simulink model "motion_with_control_two_robots"  (R2025a)
settings: Solver=FixedStepDiscrete  StartTime=0.0  StopTime=inf  FixedStep=0.01  RelTol=1e-3  EnableMultiTasking=on
PreLoadFcn:
  | frs = FrankaRobotSettings;
libraries: franka_simulink x2
settings Model: SimulationMode=external  ExtModeTrigDuration=10000  Creator=vasi_ko  LastModifiedBy=kvasios
settings SolverCC: ConcurrentTasks=on  AlgebraicLoopSolver=TrustRegion  AutoInsertRateTranBlk=on
settings DataIOCC: LimitDataPoints=on  SaveFormat=Array  ReturnWorkspaceOutputs=off
settings OptimizationCC: EnhancedBackFolding=on  PassReuseOutputArgsAs=Individual arguments  ZeroExternalMemoryAtStartup=off  ZeroInternalMemoryAtStartup=off  MaxStackSize=200000  OptimizeBlockOrder=speed  DifferentSizesBufferReuse=on  OptimizationCustomize=off  EfficientTunableParamExpr=on
settings DebuggingCC: SolverPrmCheckMsg=warning  ParameterTunabilityLossMsg=error  UnconnectedInputMsg=warning  UnconnectedOutputMsg=warning  UnconnectedLineMsg=warning  SFUnexpectedBacktrackingDiag=warning  SFNoUnconditionalDefaultTransitionDiag=warning  SFExecutionAtInitializationDiag=none  ArithmeticOperatorsInVariantConditions=warning
settings HardwareCC: ProdBitPerLong=64.0  ProdLargestAtomicInteger=LongLong  ProdLargestAtomicFloat=Double  ProdLongLongMode=on  ProdHWDeviceType=ARM Compatible->ARM Cortex-A (64-bit)
settings ModelReferenceCC: EnableRefExpFcnMdlSchedulingChecks=on  PropagateSignalLabelsOutOfModel=off
settings SFSimCC: SimUseLocalCustomCode=off  MATLABDynamicMemAlloc=off  CustomCodeUndefinedFunction=UseInterfaceOnly  SimTargetLang=C++  SimDLTargetLibrary=mkl-dnn
settings RTWCC: SystemTargetFile=ert.tlc  HardwareBoard=NVIDIA Jetson  TLCOptions="-aInlineSetEventsForThisBaseRateFcn=TLC_FALSE -aSuppressMultiTaskScheduler=TLC_FALSE  -aRateBasedStepFcn=0"  TemplateMakefile=ert_default_tmf  RTWVerbose=off  RTWUseLocalCustomCode=off  BuildConfiguration=Faster Runs  TargetLang=C++  GPUComputeCapability=3.5  DLArmComputeVersion=19.05  Description=Embedded Coder
settings CodeAppCC: ForceParamTrailComments=on  IgnoreCustomStorageClasses=off  OperatorAnnotations=on  SimulinkDataObjDesc=on  SFDataObjDesc=on  InsertBlockDesc=on
settings ERTTargetCC: ExtModeTransport=2.0  InlinedParameterPlacement=Hierarchical  RootIOFormat=Structure reference  TargetLangStandard=C++14 (ISO)
settings ConfigComp: CovMetricSettings=dw  CovSaveCumulativeToWorkspaceVar=on  CovSaveSingleToWorkspaceVar=on  CovExternalEMLEnable=off  CovSFcnEnable=off

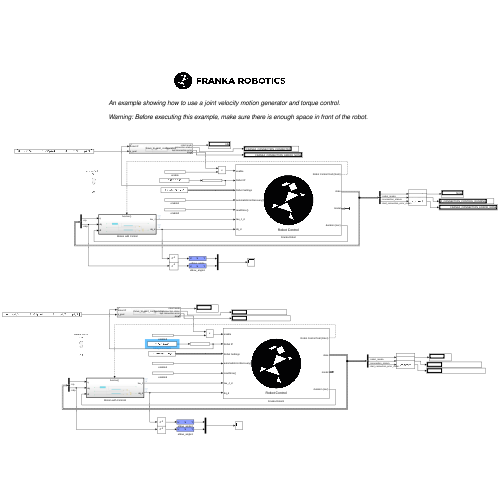
[thumbnail: Simulink's stored preview of the top-level diagram]
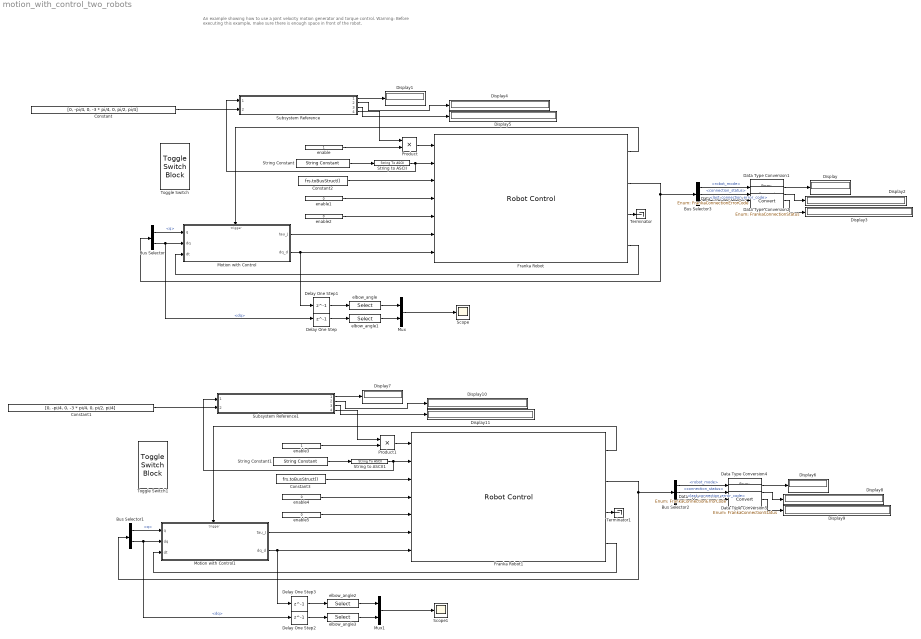
== system motion_with_control_two_robots ==
  note: An example showing how to use a joint velocity motion generator and torque control.
      |
      | Warning: Before executing this example, make sure there is enough space in front of the robot.
  Bus Selector : BusSelector  OutputSignals=q,dq
  Bus Selector1 : BusSelector  OutputSignals=q,dq
  Bus Selector2 : BusSelector  OutputSignals=robot_mode,connection_status,last_connection_error_code
  Bus Selector3 : BusSelector  OutputSignals=robot_mode,connection_status,last_connection_error_code
  Constant : Constant  Value=[0, -pi/4, 0, -3 * pi/4, 0, pi/2, pi/4]
  Constant1 : Constant  Value=[0, -pi/4, 0, -3 * pi/4, 0, pi/2, pi/4]
  Constant2 : Constant  Value=frs.toBusStruct()  OutDataTypeStr=Bus: FrankaRobotSettingsBus
  Constant3 : Constant  Value=frs.toBusStruct()  OutDataTypeStr=Bus: FrankaRobotSettingsBus
  Data Type Conversion1 : DataTypeConversion  OutDataTypeStr=Enum: FrankaRobotModes  SaturateOnIntegerOverflow=off  RndMeth=Floor
  Data Type Conversion2 : DataTypeConversion  OutDataTypeStr=Enum: FrankaConnectionStatus  SaturateOnIntegerOverflow=off  RndMeth=Floor
  Data Type Conversion3 : DataTypeConversion  OutDataTypeStr=Enum: FrankaConnectionErrorCode  SaturateOnIntegerOverflow=off  RndMeth=Floor
  Data Type Conversion4 : DataTypeConversion  OutDataTypeStr=Enum: FrankaRobotModes  SaturateOnIntegerOverflow=off  RndMeth=Floor
  Data Type Conversion5 : DataTypeConversion  OutDataTypeStr=Enum: FrankaConnectionStatus  SaturateOnIntegerOverflow=off  RndMeth=Floor
  Data Type Conversion6 : DataTypeConversion  OutDataTypeStr=Enum: FrankaConnectionErrorCode  SaturateOnIntegerOverflow=off  RndMeth=Floor
  Delay One Step{,1..3} (4 alike) : Delay  DelayLength=1
  Display{,1..11} (12 alike) : Display
  Franka Robot : franka_simulink/Robot Control  control_mode=Torques + Joint Velocities  rt_priority=80  rt_cpu_affinity=-1  rt_lock_memory=off
      settings: SourceProductName=Franka Robotics Simulink Support Package
  Franka Robot1 : franka_simulink/Robot Control  control_mode=Torques + Joint Velocities  rt_priority=80  rt_cpu_affinity=-1  rt_lock_memory=off
      settings: SourceProductName=Franka Robotics Simulink Support Package
  Motion with Control : Subsystem  TreatAsAtomicUnit=on
      settings: RTWSystemCode=Nonreusable function
  Motion with Control1 : Subsystem  TreatAsAtomicUnit=on
      settings: RTWSystemCode=Nonreusable function
  Mux : Mux  Inputs=2
  Mux1 : Mux  Inputs=2
  Product : Product
  Product1 : Product
  Scope : Scope
      settings: ActiveDisplayYMinimum=-0.68593897081558164  ActiveDisplayYMaximum=0.68922481990277773
  Scope1 : Scope
      settings: ActiveDisplayYMinimum=-0.68593897081558164  ActiveDisplayYMaximum=0.68922481990277773
  String Constant : StringConstant  String="\"172.16.0.2\""
  String Constant1 : StringConstant  String="\"172.16.0.3\""
  String to ASCII : StringToASCII  OutputVectorSize=16
  String to ASCII1 : StringToASCII  OutputVectorSize=16
  Subsystem Reference : Subsystem  ReferencedSubsystem=move_to_joint_configuration
  Subsystem Reference1 : Subsystem  ReferencedSubsystem=move_to_joint_configuration
  Terminator : Terminator
  Terminator1 : Terminator
  Toggle Switch : ToggleSwitchBlock
  Toggle Switch1 : ToggleSwitchBlock
  elbow_angle{,1..3} (4 alike) : Selector  InputPortWidth=7  IndexOptions=Index vector (dialog)  Indices=4  OutputSizes=1
  enable : Constant  SampleTime=-1
  enable{1..2,4..5} (4 alike) : Constant  Value=0  SampleTime=-1
  enable3 : Constant  SampleTime=-1
  wires:
  String to ASCII/1 -> Subsystem Reference/1, Franka Robot/2
  String Constant/1 -> String to ASCII/1
  Franka Robot/1 -> Motion with Control/Trigger
  Bus Selector/1 -> Motion with Control/1(q)  "<q>"
  Bus Selector/2 -> Delay One Step/1, Motion with Control/2(dq)  "<dq>"
  Franka Robot/4 -> Motion with Control/3(dt)
  Franka Robot/3 -> Terminator/1
  Constant2/1 -> Franka Robot/3
  Product/1 -> Franka Robot/1
  enable/1 -> Product/2
  Motion with Control/1(tau_J) -> Franka Robot/6
  enable1/1 -> Franka Robot/4
  enable2/1 -> Franka Robot/5
  Subsystem Reference/1 -> Display1/1
  Motion with Control/2(dq_d) -> Delay One Step1/1, Franka Robot/7
  elbow_angle/1 -> Mux/1
  elbow_angle1/1 -> Mux/2
  Mux/1 -> Scope/1
  Delay One Step/1 -> elbow_angle1/1
  Delay One Step1/1 -> elbow_angle/1
  Constant/1 -> Subsystem Reference/2
  Subsystem Reference/4 -> Product/1
  Subsystem Reference/2 -> Display4/1
  Subsystem Reference/3 -> Display5/1
  Bus Selector3/2 -> Data Type Conversion2/1  "<connection_status>"
  Data Type Conversion1/1 -> Display/1
  Franka Robot/2 -> Bus Selector3/1, Bus Selector/1
  Bus Selector3/1 -> Data Type Conversion1/1  "<robot_mode>"
  Data Type Conversion3/1 -> Display3/1
  Data Type Conversion2/1 -> Display2/1
  Bus Selector3/3 -> Data Type Conversion3/1  "<last_connection_error_code>"
  Bus Selector2/3 -> Data Type Conversion6/1  "<last_connection_error_code>"
  Data Type Conversion5/1 -> Display8/1
  Data Type Conversion6/1 -> Display9/1
  Bus Selector2/1 -> Data Type Conversion4/1  "<robot_mode>"
  Franka Robot1/2 -> Bus Selector1/1, Bus Selector2/1
  Data Type Conversion4/1 -> Display6/1
  Bus Selector2/2 -> Data Type Conversion5/1  "<connection_status>"
  Subsystem Reference1/3 -> Display11/1
  Subsystem Reference1/2 -> Display10/1
  Subsystem Reference1/4 -> Product1/1
  Constant1/1 -> Subsystem Reference1/2
  Delay One Step3/1 -> elbow_angle2/1
  Delay One Step2/1 -> elbow_angle3/1
  Mux1/1 -> Scope1/1
  elbow_angle3/1 -> Mux1/2
  elbow_angle2/1 -> Mux1/1
  Motion with Control1/2(dq_d) -> Franka Robot1/7, Delay One Step3/1
  Subsystem Reference1/1 -> Display7/1
  enable5/1 -> Franka Robot1/5
  enable4/1 -> Franka Robot1/4
  Motion with Control1/1(tau_J) -> Franka Robot1/6
  enable3/1 -> Product1/2
  Product1/1 -> Franka Robot1/1
  Constant3/1 -> Franka Robot1/3
  Franka Robot1/3 -> Terminator1/1
  Franka Robot1/4 -> Motion with Control1/3(dt)
  Bus Selector1/2 -> Motion with Control1/2(dq), Delay One Step2/1  "<dq>"
  Bus Selector1/1 -> Motion with Control1/1(q)  "<q>"
  Franka Robot1/1 -> Motion with Control1/Trigger
  String Constant1/1 -> String to ASCII1/1
  String to ASCII1/1 -> Franka Robot1/2, Subsystem Reference1/1

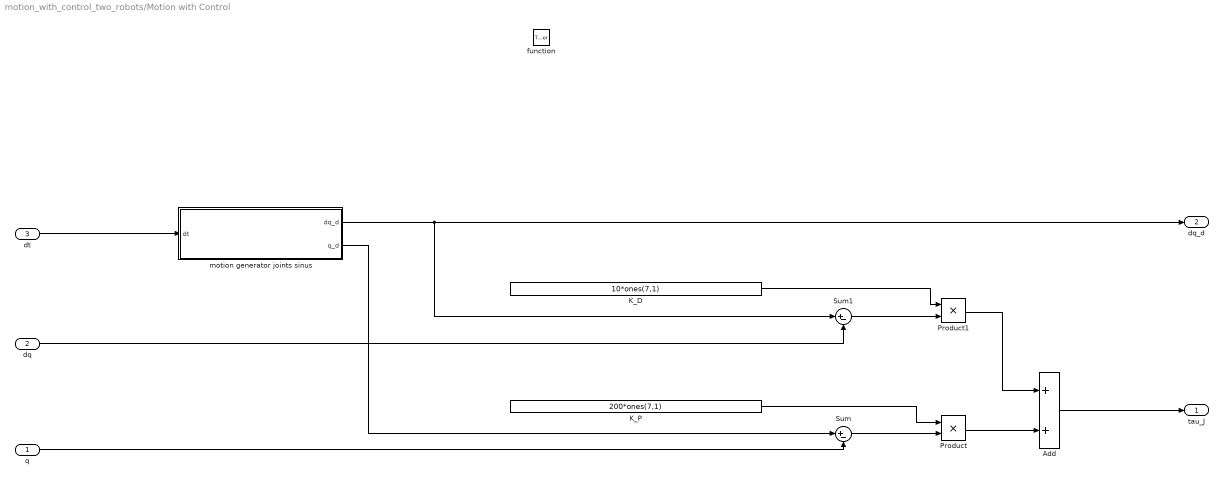
== system motion_with_control_two_robots/Motion with Control ==
  q : Inport
  dq : Inport  Port=2
  dt : Inport  Port=3
  function : TriggerPort  TriggerType=function-call  VariantControl=(inherit)  SampleTime=0.001
  Add : Sum
  K_D : Constant  Value=10*ones(7,1)  VectorParams1D=off  SampleTime=-1
  K_P : Constant  Value=200*ones(7,1)  VectorParams1D=off  SampleTime=-1
  Product : Product
  Product1 : Product
  Sum : Sum  Inputs=|+-
  Sum1 : Sum  Inputs=|+-
  motion generator joints sinus : Subsystem
      mask Display:
      | pos = get_param(gcb, 'Position');
      | width = pos(3) - pos(1);
      | x = [0:width];
      | y = sin(x/180*pi);
      | % Parameters 'm' and 'b' must be defined in 'Parameters & Dialog' pane.
      | plot(x,y );
      | 
      | port_label('output',1,'dq_d');
      | port_label('output',2,'q_d');
  tau_J : Outport  VectorParamsAs1DForOutWhenUnconnected=off
  dq_d : Outport  Port=2  VectorParamsAs1DForOutWhenUnconnected=off
  wires:
  Product1/1 -> Add/1
  Sum1/1 -> Product1/2
  dq/1 -> Sum1/2
  Product/1 -> Add/2
  Sum/1 -> Product/2
  K_D/1 -> Product1/1
  q/1 -> Sum/2
  K_P/1 -> Product/1
  dt/1 -> motion generator joints sinus/1(dt)
  motion generator joints sinus/1(dq_d) -> dq_d/1, Sum1/1
  motion generator joints sinus/2(q_d) -> Sum/1
  Add/1 -> tau_J/1

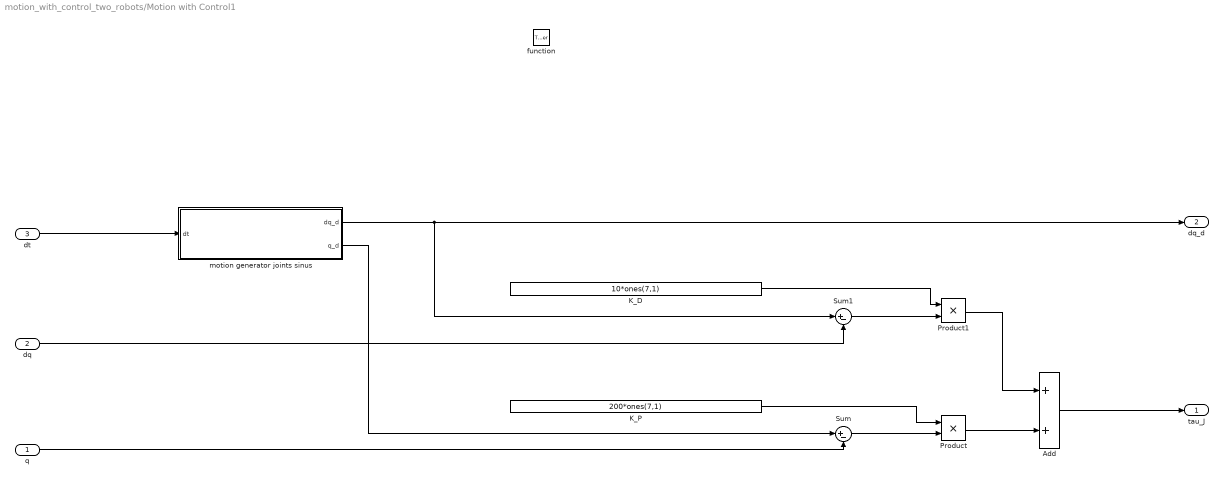
== system motion_with_control_two_robots/Motion with Control1 ==
  q : Inport
  dq : Inport  Port=2
  dt : Inport  Port=3
  function : TriggerPort  TriggerType=function-call  VariantControl=(inherit)  SampleTime=0.001
  Add : Sum
  K_D : Constant  Value=10*ones(7,1)  VectorParams1D=off  SampleTime=-1
  K_P : Constant  Value=200*ones(7,1)  VectorParams1D=off  SampleTime=-1
  Product : Product
  Product1 : Product
  Sum : Sum  Inputs=|+-
  Sum1 : Sum  Inputs=|+-
  motion generator joints sinus : Subsystem
      mask Display:
      | pos = get_param(gcb, 'Position');
      | width = pos(3) - pos(1);
      | x = [0:width];
      | y = sin(x/180*pi);
      | % Parameters 'm' and 'b' must be defined in 'Parameters & Dialog' pane.
      | plot(x,y );
      | 
      | port_label('output',1,'dq_d');
      | port_label('output',2,'q_d');
  tau_J : Outport  VectorParamsAs1DForOutWhenUnconnected=off
  dq_d : Outport  Port=2  VectorParamsAs1DForOutWhenUnconnected=off
  wires:
  Add/1 -> tau_J/1
  motion generator joints sinus/2(q_d) -> Sum/1
  motion generator joints sinus/1(dq_d) -> Sum1/1, dq_d/1
  dt/1 -> motion generator joints sinus/1(dt)
  K_P/1 -> Product/1
  q/1 -> Sum/2
  K_D/1 -> Product1/1
  Sum/1 -> Product/2
  Product/1 -> Add/2
  dq/1 -> Sum1/2
  Sum1/1 -> Product1/2
  Product1/1 -> Add/1

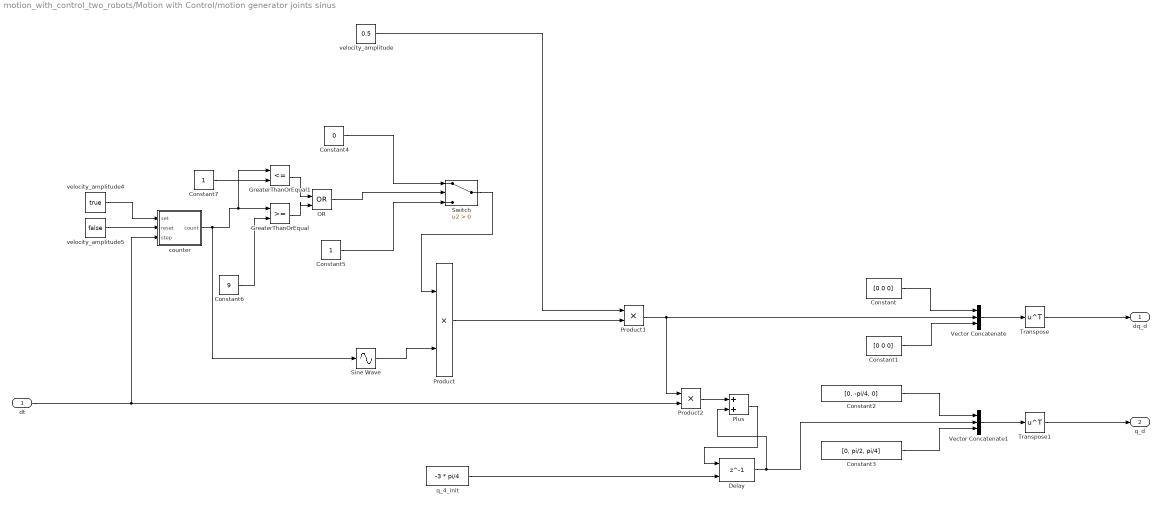
== system motion_with_control_two_robots/Motion with Control/motion generator joints sinus ==
  dt : Inport
  Constant : Constant  Value=[0 0 0]  VectorParams1D=off
  Constant1 : Constant  Value=[0 0 0]  VectorParams1D=off
  Constant2 : Constant  Value=[0, -pi/4, 0]  VectorParams1D=off
  Constant3 : Constant  Value=[0, pi/2, pi/4]  VectorParams1D=off
  Constant4 : Constant  Value=0
  Constant5 : Constant
  Constant6 : Constant  Value=9
  Constant7 : Constant
  Delay : Delay  DelayLength=1  InitialConditionSource=Input port
      settings: InputPortMap=u0,p4
  GreaterThanOrEqual : RelationalOperator  OutDataTypeStr=boolean  RndMeth=Simplest  InputSameDT=off
  GreaterThanOrEqual1 : RelationalOperator  Operator=<=  OutDataTypeStr=boolean  RndMeth=Simplest  InputSameDT=off
  OR : Logic  Operator=OR  IconShape=distinctive  AllPortsSameDT=off  OutDataTypeStr=boolean
  Plus : Sum
  Product : Product
  Product1 : Product
  Product2 : Product
  Sine Wave : Sin  TimeSource=Use external signal  Frequency=pi  Phase=pi
  Switch : Switch  Criteria=u2 > Threshold  SaturateOnIntegerOverflow=off  InputSameDT=off
  Transpose : Math  Operator=transpose
  Transpose1 : Math  Operator=transpose
  Vector Concatenate : Concatenate  NumInputs=3
  Vector Concatenate1 : Concatenate  NumInputs=3
  counter : Subsystem
  q_4_init : Constant  Value=-3 * pi/4  VectorParams1D=off
  velocity_amplitude : Constant  Value=0.5  VectorParams1D=off
  velocity_amplitude4 : Constant  Value=true  VectorParams1D=off
  velocity_amplitude5 : Constant  Value=false  VectorParams1D=off
  dq_d : Outport  VectorParamsAs1DForOutWhenUnconnected=off
  q_d : Outport  Port=2  VectorParamsAs1DForOutWhenUnconnected=off
  wires:
  Constant1/1 -> Vector Concatenate/3
  Constant/1 -> Vector Concatenate/1
  Product/1 -> Product1/2
  Sine Wave/1 -> Product/2
  velocity_amplitude/1 -> Product1/1
  Product1/1 -> Vector Concatenate/2, Product2/1
  Constant3/1 -> Vector Concatenate1/3
  Constant2/1 -> Vector Concatenate1/1
  q_4_init/1 -> Delay/2
  Delay/1 -> Vector Concatenate1/2, Plus/2
  Plus/1 -> Delay/1
  Product2/1 -> Plus/1
  Vector Concatenate/1 -> Transpose/1
  Vector Concatenate1/1 -> Transpose1/1
  Transpose/1 -> dq_d/1
  Transpose1/1 -> q_d/1
  velocity_amplitude4/1 -> counter/1(set)
  velocity_amplitude5/1 -> counter/2(reset)
  dt/1 -> counter/3(step), Product2/2
  Constant4/1 -> Switch/1
  Constant5/1 -> Switch/3
  Constant6/1 -> GreaterThanOrEqual/2
  Switch/1 -> Product/1
  GreaterThanOrEqual1/1 -> OR/1
  GreaterThanOrEqual/1 -> OR/2
  OR/1 -> Switch/2
  counter/1(count) -> Sine Wave/1, GreaterThanOrEqual1/1, GreaterThanOrEqual/1
  Constant7/1 -> GreaterThanOrEqual1/2

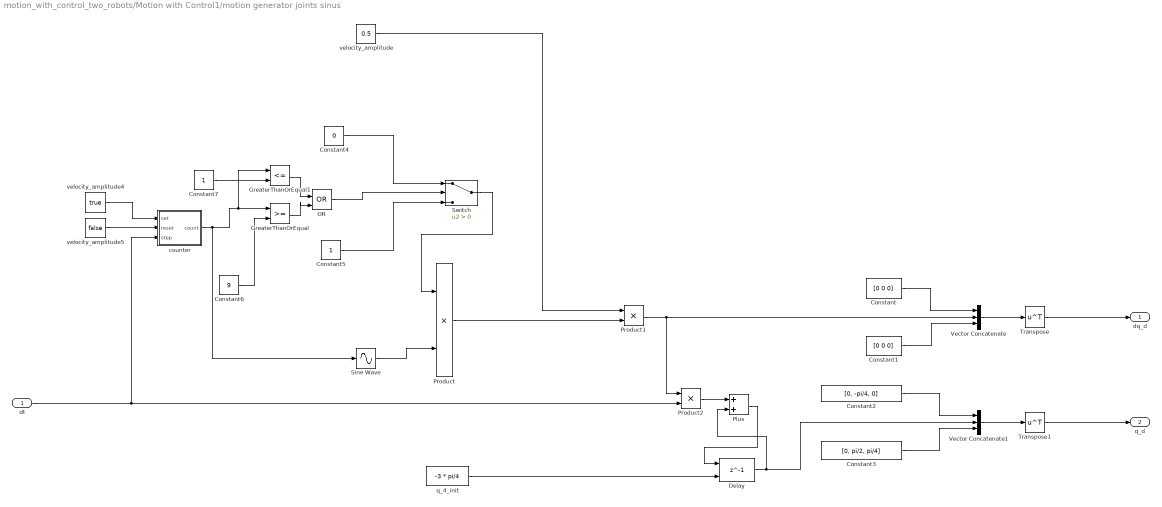
== system motion_with_control_two_robots/Motion with Control1/motion generator joints sinus ==
  dt : Inport
  Constant : Constant  Value=[0 0 0]  VectorParams1D=off
  Constant1 : Constant  Value=[0 0 0]  VectorParams1D=off
  Constant2 : Constant  Value=[0, -pi/4, 0]  VectorParams1D=off
  Constant3 : Constant  Value=[0, pi/2, pi/4]  VectorParams1D=off
  Constant4 : Constant  Value=0
  Constant5 : Constant
  Constant6 : Constant  Value=9
  Constant7 : Constant
  Delay : Delay  DelayLength=1  InitialConditionSource=Input port
      settings: InputPortMap=u0,p4
  GreaterThanOrEqual : RelationalOperator  OutDataTypeStr=boolean  RndMeth=Simplest  InputSameDT=off
  GreaterThanOrEqual1 : RelationalOperator  Operator=<=  OutDataTypeStr=boolean  RndMeth=Simplest  InputSameDT=off
  OR : Logic  Operator=OR  IconShape=distinctive  AllPortsSameDT=off  OutDataTypeStr=boolean
  Plus : Sum
  Product : Product
  Product1 : Product
  Product2 : Product
  Sine Wave : Sin  TimeSource=Use external signal  Frequency=pi  Phase=pi
  Switch : Switch  Criteria=u2 > Threshold  SaturateOnIntegerOverflow=off  InputSameDT=off
  Transpose : Math  Operator=transpose
  Transpose1 : Math  Operator=transpose
  Vector Concatenate : Concatenate  NumInputs=3
  Vector Concatenate1 : Concatenate  NumInputs=3
  counter : Subsystem
  q_4_init : Constant  Value=-3 * pi/4  VectorParams1D=off
  velocity_amplitude : Constant  Value=0.5  VectorParams1D=off
  velocity_amplitude4 : Constant  Value=true  VectorParams1D=off
  velocity_amplitude5 : Constant  Value=false  VectorParams1D=off
  dq_d : Outport  VectorParamsAs1DForOutWhenUnconnected=off
  q_d : Outport  Port=2  VectorParamsAs1DForOutWhenUnconnected=off
  wires:
  Constant7/1 -> GreaterThanOrEqual1/2
  counter/1(count) -> GreaterThanOrEqual/1, GreaterThanOrEqual1/1, Sine Wave/1
  OR/1 -> Switch/2
  GreaterThanOrEqual/1 -> OR/2
  GreaterThanOrEqual1/1 -> OR/1
  Switch/1 -> Product/1
  Constant6/1 -> GreaterThanOrEqual/2
  Constant5/1 -> Switch/3
  Constant4/1 -> Switch/1
  dt/1 -> Product2/2, counter/3(step)
  velocity_amplitude5/1 -> counter/2(reset)
  velocity_amplitude4/1 -> counter/1(set)
  Transpose1/1 -> q_d/1
  Transpose/1 -> dq_d/1
  Vector Concatenate1/1 -> Transpose1/1
  Vector Concatenate/1 -> Transpose/1
  Product2/1 -> Plus/1
  Plus/1 -> Delay/1
  Delay/1 -> Plus/2, Vector Concatenate1/2
  q_4_init/1 -> Delay/2
  Constant2/1 -> Vector Concatenate1/1
  Constant3/1 -> Vector Concatenate1/3
  Product1/1 -> Product2/1, Vector Concatenate/2
  velocity_amplitude/1 -> Product1/1
  Sine Wave/1 -> Product/2
  Product/1 -> Product1/2
  Constant/1 -> Vector Concatenate/1
  Constant1/1 -> Vector Concatenate/3

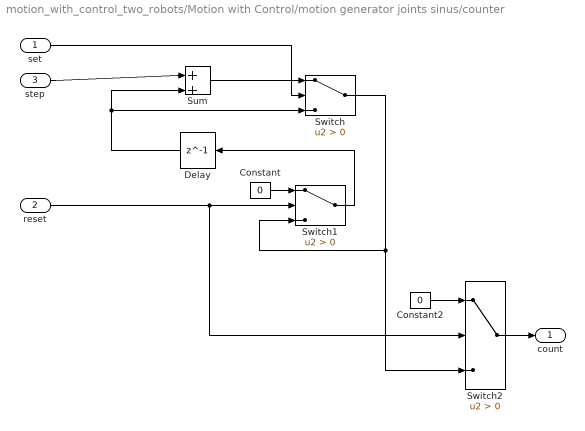
== system motion_with_control_two_robots/Motion with Control/motion generator joints sinus/counter ==
  set : Inport  OutDataTypeStr=boolean
  reset : Inport  Port=2  OutDataTypeStr=boolean
  step : Inport  Port=3  OutDataTypeStr=double
  Constant : Constant  Value=0  OutDataTypeStr=double
  Constant2 : Constant  Value=0  OutDataTypeStr=double
  Delay : Delay  DelayLength=1  InitialCondition=0
  Sum : Sum  Inputs=|++
  Switch : Switch  Criteria=u2 > Threshold  SaturateOnIntegerOverflow=off  InputSameDT=off
  Switch1 : Switch  Criteria=u2 > Threshold  OutDataTypeStr=double  SaturateOnIntegerOverflow=off  InputSameDT=off
  Switch2 : Switch  Criteria=u2 > Threshold  OutDataTypeStr=double  SaturateOnIntegerOverflow=off  InputSameDT=off
  count : Outport  OutDataTypeStr=double  VectorParamsAs1DForOutWhenUnconnected=off
  wires:
  Switch2/1 -> count/1
  Constant2/1 -> Switch2/1
  Sum/1 -> Switch/1
  set/1 -> Switch/2
  Switch/1 -> Switch1/3, Switch2/3
  step/1 -> Sum/1
  Delay/1 -> Sum/2, Switch/3
  reset/1 -> Switch1/2, Switch2/2
  Constant/1 -> Switch1/1
  Switch1/1 -> Delay/1

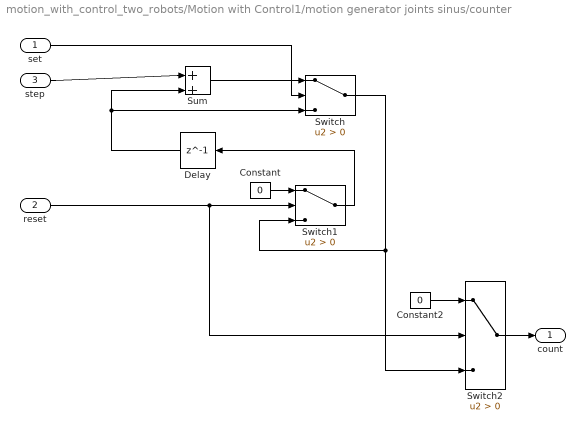
== system motion_with_control_two_robots/Motion with Control1/motion generator joints sinus/counter ==
  set : Inport  OutDataTypeStr=boolean
  reset : Inport  Port=2  OutDataTypeStr=boolean
  step : Inport  Port=3  OutDataTypeStr=double
  Constant : Constant  Value=0  OutDataTypeStr=double
  Constant2 : Constant  Value=0  OutDataTypeStr=double
  Delay : Delay  DelayLength=1  InitialCondition=0
  Sum : Sum  Inputs=|++
  Switch : Switch  Criteria=u2 > Threshold  SaturateOnIntegerOverflow=off  InputSameDT=off
  Switch1 : Switch  Criteria=u2 > Threshold  OutDataTypeStr=double  SaturateOnIntegerOverflow=off  InputSameDT=off
  Switch2 : Switch  Criteria=u2 > Threshold  OutDataTypeStr=double  SaturateOnIntegerOverflow=off  InputSameDT=off
  count : Outport  OutDataTypeStr=double  VectorParamsAs1DForOutWhenUnconnected=off
  wires:
  Switch1/1 -> Delay/1
  Constant/1 -> Switch1/1
  reset/1 -> Switch2/2, Switch1/2
  Delay/1 -> Switch/3, Sum/2
  step/1 -> Sum/1
  Switch/1 -> Switch2/3, Switch1/3
  set/1 -> Switch/2
  Sum/1 -> Switch/1
  Constant2/1 -> Switch2/1
  Switch2/1 -> count/1
